simulink model "MOCS_AS_Gen"  (R2024b)
settings: Solver=FixedStepDiscrete  StartTime=0.0  StopTime=inf  FixedStep=SamplingTime  RelTol=1e-3
PostLoadFcn:
  | init_EXT_SRTUCT_IN;
model workspace: external: MAT-File (data not in the file)
undefined symbols (not defined in the file): IF_MATIN_IO, IF_PARA, IO_typ, Para_typ, Tick_100ms
libraries: simulink x10, bur_blks x3, Lib_Model x1
settings Model: DataDictionary=mainDB.sldd  Creator=HHI  LastModifiedBy=HHI
settings DataIOCC: SaveFormat=Array  SaveOutput=off  SignalLogging=off  DSMLogging=off  SaveTime=off  ReturnWorkspaceOutputs=off
settings OptimizationCC: ReuseModelBlockBuffer=off  EnableMemcpy=off  ZeroExternalMemoryAtStartup=off  ZeroInternalMemoryAtStartup=off  InitFltsAndDblsToZero=on  LifeSpan=inf  OptimizeBlockOrder=speed  DifferentSizesBufferReuse=on  EfficientTunableParamExpr=on
settings DebuggingCC: UnderspecifiedInitializationDetection=Classic  MergeDetectMultiDrivingBlocksExec=none  SolverPrmCheckMsg=warning  InheritedTsInSrcMsg=none  FcnCallInpInsideContextMsg=warning  UnconnectedInputMsg=warning  UnconnectedOutputMsg=warning  UnconnectedLineMsg=warning  FrameProcessingCompatibilityMsg=none  ModelReferenceSymbolNameMessage=none  StateNameClashWarn=warning  SFUnexpectedBacktrackingDiag=warning  SFNoUnconditionalDefaultTransitionDiag=warning
settings HardwareCC: ProdBitPerPointer=32  ProdBitPerSizeT=32  ProdBitPerPtrDiffT=32  ProdLargestAtomicFloat=None  ProdWordSize=32  ProdHWDeviceType=Intel->x86/Pentium
settings ModelReferenceCC: UpdateModelReferenceTargets=IfOutOfDate  ModelReferencePassRootInputsByReference=off  PropagateSignalLabelsOutOfModel=off
settings SFSimCC: MATLABDynamicMemAlloc=off
settings RTWCC: Description=B&R Automation Studio Target (ERT based)  SystemTargetFile=bur_ert.tlc  GenCodeOnly=on  GenerateMakefile=off  TemplateMakefile=bur.tmf  RTWVerbose=off  GPUComputeCapability=3.5
settings CodeAppCC: IgnoreTestpoints=on  CustomSymbolStrType=$N$R$M  InternalIdentifier=Classic
settings STFCustomTargetCC: TargetLangStandard=C99 (ISO)  MultiwordLength=256  ParMdlRefBuildCompliant=on  ERTCustomFileBanners=on  SupportNonFinite=off  SupportNonInlinedSFcns=off  RemoveResetFunc=on  MATLABClassNameForMDSCustomization=Simulink.SoftwareTarget.ERTCustomization  SystemTargetFile=bur_ert.tlc
settings ERTTargetCC: TargetLangStandard=C99 (ISO)  CompOptLevelCompliant=off  ConcurrentExecutionCompliant=off  CombineOutputUpdateFcns=off  SupportNonFinite=off  SupportContinuousTime=on  ModelStepFunctionPrototypeControlCompliant=off  CPPClassGenCompliant=off  UseToolchainInfoCompliant=off  ExtModeMexArgs='127.0.0.1'  InlinedParameterPlacement=Hierarchical  MultiInstanceErrorCode=Warning  RootIOFormat=Structure reference  ERTSrcFileBannerTemplate=bur_code_c_template.cgt  ERTHdrFileBannerTemplate=bur_code_h_template.cgt  ERTDataSrcFileTemplate=bur_data_c_template.cgt  ERTDataHdrFileTemplate=bur_data_h_template.cgt  ERTCustomFileTemplate=bur_file_process.tlc  ConvertIfToSwitch=off  SuppressUnreachableDefaultCases=off  DynamicArrayContainerType=coder::array

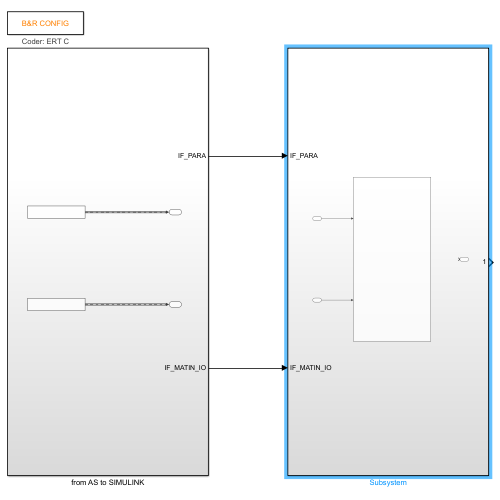
[thumbnail: Simulink's stored preview of the top-level diagram]
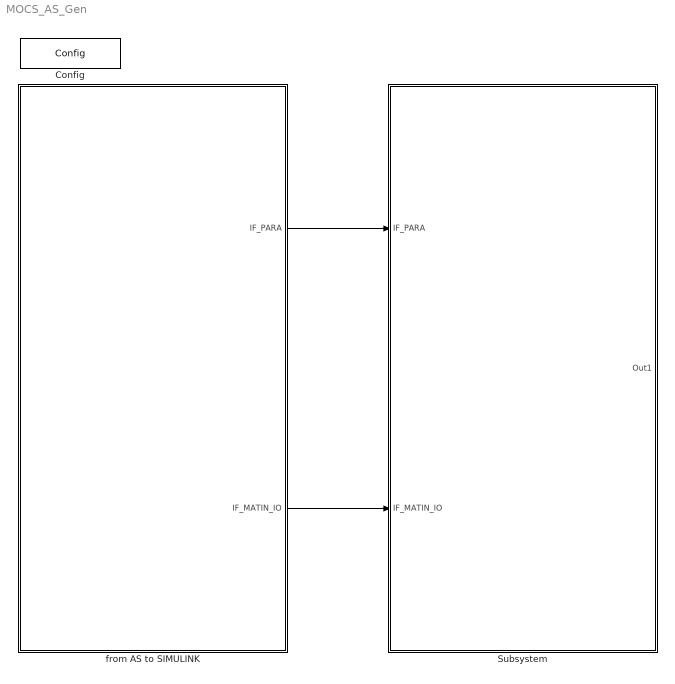
== system MOCS_AS_Gen ==
  Config : bur_blks/Config  Tag=Coder: ERT C Target: Task  bur_configset_ert=C - Code Generation (Embedded Real Time Target based)  bur_configset_grt=C - Code Generation (Generic Real Time Target based)  bur_maskHandle=-1
      settings: AttributesFormatString=%<Tag>  SourceProductName=B&R Automation Studio Toolbox
  Subsystem : Subsystem
  from AS to SIMULINK : Subsystem
  wires:
  from AS to SIMULINK/1(IF_PARA) -> Subsystem/1(IF_PARA)
  from AS to SIMULINK/2(IF_MATIN_IO) -> Subsystem/2(IF_MATIN_IO)

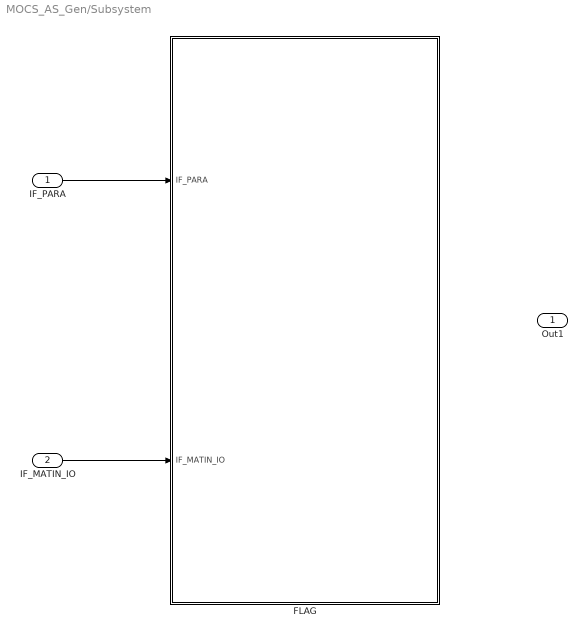
== system MOCS_AS_Gen/Subsystem ==
  IF_PARA : Inport
  IF_MATIN_IO : Inport  Port=2
  FLAG : Subsystem
  Out1 : Outport
  wires:
  IF_PARA/1 -> FLAG/1(IF_PARA)
  IF_MATIN_IO/1 -> FLAG/2(IF_MATIN_IO)

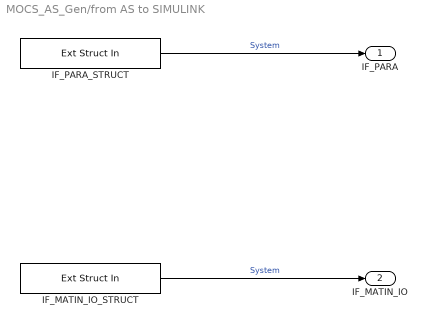
== system MOCS_AS_Gen/from AS to SIMULINK ==
  IF_MATIN_IO_STRUCT : bur_blks/Ext Struct In  Tag=GLOBAL IO_typ IF_MATIN_IO  bur_var_name=IF_MATIN_IO  bur_scope=GLOBAL  bur_var_memory=standard  bur_struct_name=IO_typ  bur_AS_string=IF_MATIN_IO : IO_typ; (**)  bur_AS_typ_list_string=|
      | IO_typ
      | Bus: CommIO_typ
      | Bus: CommMOCSIO_typ
      | Bus: CMDI_typ
      | Bus: CMDO_typ
      | Bus: CommFODSIO_typ
      | Bus: CFAI_typ
      | Bus: CFDI_typ
      | Bus: CFDO_typ
      | Bus: IndivIO_typ
      | Bus: IndivMOCSIO_typ
      | Bus: IMAI_typ
      | Bus: IMAO_typ
      | Bus: IMDI_typ
      | Bus: IMDO_typ
      | Bus: IndivFODSIO_typ
      | Bus: IFAI_typ
      | Bus: IFAO_typ
      | Bus: IFDI_typ
      | Bus: IFDO_typ
      | Bus: IndivSCRIO_typ
      | Bus: ISDI_typ
      | Bus: ISDO_typ
      | Bus: IndivIO_typ
      | Bus: IndivMOCSIO_typ
      | Bus: IMAI_typ
      | Bus: IMAO_typ
      | Bus: IMDI_typ
      | Bus: IMDO_typ
      | Bus: IndivFODSIO_typ
      | Bus: IFAI_typ
      | Bus: IFAO_typ
      | Bus: IFDI_typ
      | Bus: IFDO_typ
      | Bus: IndivSCRIO_typ
      | Bus: ISDI_typ
      | Bus: ISDO_typ
      | Bus: IndivIO_typ
      | Bus: IndivMOCSIO_typ
      | Bus: IMAI_typ
      | Bus: IMAO_typ
      | Bus: IMDI_typ
      | Bus: IMDO_typ
      | Bus: IndivFODSIO_typ
      | Bus: IFAI_typ
      | Bus: IFAO_typ
      | Bus: IFDI_typ
      | Bus: IFDO_typ
      | Bus: IndivSCRIO_typ
      | Bus: ISDI_typ
      | Bus: ISDO_typ
      | Bus: IndivIO_typ
      | Bus: IndivMOCSIO_typ
      | Bus: IMAI_typ
      | Bus: IMAO_typ
      | Bus: IMDI_typ
      | Bus: IMDO_typ
      | Bus: IndivFODSIO_typ
      | Bus: IFAI_typ
      | Bus: IFAO_typ
      | Bus: IFDI_typ
      | Bus: IFDO_typ
      | Bus: IndivSCRIO_typ
      | Bus: ISDI_typ
      | Bus: ISDO_typ
      | Bus: IndivIO_typ
      | Bus: IndivMOCSIO_typ
      | Bus: IMAI_typ
      | Bus: IMAO_typ
      | Bus: IMDI_typ
      | Bus: IMDO_typ
      | Bus: IndivFODSIO_typ
      | Bus: IFAI_typ
      | Bus: IFAO_typ
      | Bus: IFDI_typ
      | Bus: IFDO_typ
      | Bus: IndivSCRIO_typ
      | Bus: ISDI_typ
      | Bus: ISDO_typ
      | Bus: IndivIO_typ
      | Bus: IndivMOCSIO_typ
      | Bus: IMAI_typ
      | Bus: IMAO_typ
      | Bus: IMDI_typ
      | Bus: IMDO_typ
      | Bus: IndivFODSIO_typ
      | Bus: IFAI_typ
      | Bus: IFAO_typ
      | Bus: IFDI_typ
      | Bus: IFDO_typ
      | Bus: IndivSCRIO_typ
      | Bus: ISDI_typ
      | Bus: ISDO_typ
      | Bus: IndivIO_typ
      | Bus: IndivMOCSIO_typ
      | Bus: IMAI_typ
      | Bus: IMAO_typ
      | Bus: IMDI_typ
      | Bus: IMDO_typ
      | Bus: IndivFODSIO_typ
      | Bus: IFAI_typ
      | Bus: IFAO_typ
      | Bus: IFDI_typ
      | Bus: IFDO_typ
      | Bus: IndivSCRIO_typ
      | Bus: ISDI_typ
      | Bus: ISDO_typ
      | Bus: IndivIO_typ
      | Bus: IndivMOCSIO_typ
      | Bus: IMAI_typ
      | Bus: IMAO_typ
      | Bus: IMDI_typ
      | Bus: IMDO_typ
      | Bus: IndivFODSIO_typ
      | Bus: IFAI_typ
      | Bus: IFAO_typ
      | Bus: IFDI_typ
      | Bus: IFDO_typ
      | Bus: IndivSCRIO_typ
      | Bus: ISDI_typ
      | Bus: ISDO_typ
      settings: AttributesFormatString=%<Tag>  SourceProductName=B&R Automation Studio Toolbox
  IF_PARA_STRUCT : bur_blks/Ext Struct In  Tag=GLOBAL Para_typ IF_PARA  bur_var_name=IF_PARA  bur_scope=GLOBAL  bur_var_memory=standard  bur_struct_name=Para_typ  bur_AS_string=IF_PARA : Para_typ; (**)  bur_AS_typ_list_string=|
      | Para_typ
      | Bus: ParaCommon_typ
      | Bus: System_typ
      | Bus: SystemType_typ
      | Bus: SystemReserved_typ
      | Bus: StateFlag_typ
      | Bus: MSSNormalFlag_typ
      | Bus: LoadChangeFlag_typ
      | Bus: SystemWarmedUpFlag_typ
      | Bus: TMBFlag_typ
      | Bus: FlagReserved_typ
      | Bus: Main_typ
      | Bus: Init_typ
      | Bus: Sealing_typ
      | Bus: Engage_typ
      | Bus: Active_typ
      | Bus: TMB_typ
      | Bus: Disengage_typ
      | Bus: Airventing_typ
      | Bus: MOCSshutdown_typ
      | Bus: Valveshutdown_typ
      | Bus: FODS_typ
      | Bus: FODSInitReady_typ
      | Bus: FODSCooling_typ
      | Bus: FODSDosing_typ
      | Bus: FODSFlushing_typ
      | Bus: CommonReservedCat2_typ
      | Bus: CommonReservedCat3_typ
      | Bus: ParaIndiv_typ
      | Bus: FODSFeedforward_typ
      | Bus: FFpara_typ
      | Bus: EngineLoad_typ
      | Bus: ExhFlowrate_typ
      | Bus: HUInletRefTemp_typ
      | Bus: CorrectionFactor_typ
      | Bus: FODSFeedback_typ
      | Bus: MOCSTempPgain_typ
      | Bus: APIDgain_typ
      | Bus: IndivReservedCat2_typ
      | Bus: IndivReservedCat3_typ
      | Bus: ParaIndiv_typ
      | Bus: FODSFeedforward_typ
      | Bus: FFpara_typ
      | Bus: EngineLoad_typ
      | Bus: ExhFlowrate_typ
      | Bus: HUInletRefTemp_typ
      | Bus: CorrectionFactor_typ
      | Bus: FODSFeedback_typ
      | Bus: MOCSTempPgain_typ
      | Bus: APIDgain_typ
      | Bus: IndivReservedCat2_typ
      | Bus: IndivReservedCat3_typ
      | Bus: ParaIndiv_typ
      | Bus: FODSFeedforward_typ
      | Bus: FFpara_typ
      | Bus: EngineLoad_typ
      | Bus: ExhFlowrate_typ
      | Bus: HUInletRefTemp_typ
      | Bus: CorrectionFactor_typ
      | Bus: FODSFeedback_typ
      | Bus: MOCSTempPgain_typ
      | Bus: APIDgain_typ
      | Bus: IndivReservedCat2_typ
      | Bus: IndivReservedCat3_typ
      | Bus: ParaIndiv_typ
      | Bus: FODSFeedforward_typ
      | Bus: FFpara_typ
      | Bus: EngineLoad_typ
      | Bus: ExhFlowrate_typ
      | Bus: HUInletRefTemp_typ
      | Bus: CorrectionFactor_typ
      | Bus: FODSFeedback_typ
      | Bus: MOCSTempPgain_typ
      | Bus: APIDgain_typ
      | Bus: IndivReservedCat2_typ
      | Bus: IndivReservedCat3_typ
      | Bus: ParaIndiv_typ
      | Bus: FODSFeedforward_typ
      | Bus: FFpara_typ
      | Bus: EngineLoad_typ
      | Bus: ExhFlowrate_typ
      | Bus: HUInletRefTemp_typ
      | Bus: CorrectionFactor_typ
      | Bus: FODSFeedback_typ
      | Bus: MOCSTempPgain_typ
      | Bus: APIDgain_typ
      | Bus: IndivReservedCat2_typ
      | Bus: IndivReservedCat3_typ
      | Bus: ParaIndiv_typ
      | Bus: FODSFeedforward_typ
      | Bus: FFpara_typ
      | Bus: EngineLoad_typ
      | Bus: ExhFlowrate_typ
      | Bus: HUInletRefTemp_typ
      | Bus: CorrectionFactor_typ
      | Bus: FODSFeedback_typ
      | Bus: MOCSTempPgain_typ
      | Bus: APIDgain_typ
      | Bus: IndivReservedCat2_typ
      | Bus: IndivReservedCat3_typ
      | Bus: ParaIndiv_typ
      | Bus: FODSFeedforward_typ
      | Bus: FFpara_typ
      | Bus: EngineLoad_typ
      | Bus: ExhFlowrate_typ
      | Bus: HUInletRefTemp_typ
      | Bus: CorrectionFactor_typ
      | Bus: FODSFeedback_typ
      | Bus: MOCSTempPgain_typ
      | Bus: APIDgain_typ
      | Bus: IndivReservedCat2_typ
      | Bus: IndivReservedCat3_typ
      | Bus: ParaIndiv_typ
      | Bus: FODSFeedforward_typ
      | Bus: FFpara_typ
      | Bus: EngineLoad_typ
      | Bus: ExhFlowrate_typ
      | Bus: HUInletRefTemp_typ
      | Bus: CorrectionFactor_typ
      | Bus: FODSFeedback_typ
      | Bus: MOCSTempPgain_typ
      | Bus: APIDgain_typ
      | Bus: IndivReservedCat2_typ
      | Bus: IndivReservedCat3_typ
      settings: AttributesFormatString=%<Tag>  SourceProductName=B&R Automation Studio Toolbox
  IF_PARA : Outport
  IF_MATIN_IO : Outport  Port=2
  wires:
  IF_MATIN_IO_STRUCT/1 -> IF_MATIN_IO/1  "System"
  IF_PARA_STRUCT/1 -> IF_PARA/1  "System"

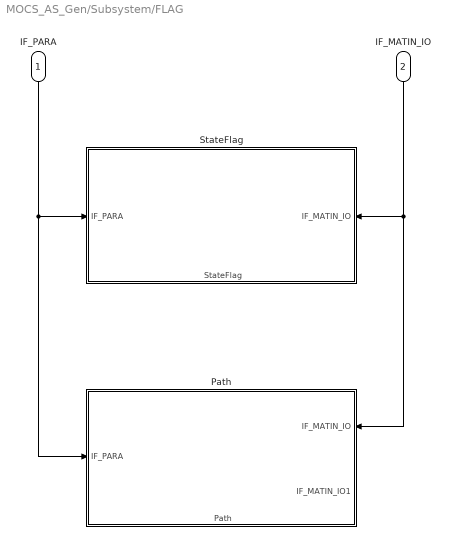
== system MOCS_AS_Gen/Subsystem/FLAG ==
  IF_PARA : Inport
  IF_MATIN_IO : Inport  Port=2
  Path : Subsystem
      settings: PortSchema="{\"entries\":[{\"content\":{\"sides\":[{\"content\":{\"connectorIds\":[\"In1\"]},\"type\":\"ConnectorPlacement.EquallySpacedRectSide\",\"uuid\":\"1f318d8d-d3a5-4a2a-9b6b-9d175d0730d5\"},{\"content\":{\"connectorIds\":[\"In2\",\"In3\"],\"side\":\"RIGHT\"},\"type\":\"ConnectorPlacement.EquallySpacedRectSide\",\"uuid\":\"3adb6d5c-76f6-48ff-b596-6c67523adb18\"},{\"content\":{\"side\":\"TOP\"},\"type\":\"ConnectorPlacement.EquallySpacedRectSide\",\"uuid\":\"8e39d891-14ef-4b5d-bc89-d43298abfc6f\"},{\"content\":{\"connectorIds\":[\"Out1\"],\"side\":\"BOTTOM\"},\"type\":\"ConnectorPlacement.EquallySpacedRectSide\",\"uuid\":\"e469beb5-ea4e-4c11-97b4-1468e014fe2c\"}]},\"type\":\"ConnectorPlacement.EquallySpacedConnector\",\"uuid\":\"bc676d84-16bc-4c83-9fee-587d58932695\"}],\"packageUris\":[\"http://schema.mathworks.com/mf0/Connector/R2020b\"],\"version\":\"1.0\"}"
  StateFlag : Subsystem
      settings: PortSchema="{\"entries\":[{\"content\":{\"sides\":[{\"content\":{\"connectorIds\":[\"In1\"]},\"type\":\"ConnectorPlacement.EquallySpacedRectSide\",\"uuid\":\"1f318d8d-d3a5-4a2a-9b6b-9d175d0730d5\"},{\"content\":{\"connectorIds\":[\"In2\"],\"side\":\"RIGHT\"},\"type\":\"ConnectorPlacement.EquallySpacedRectSide\",\"uuid\":\"3adb6d5c-76f6-48ff-b596-6c67523adb18\"},{\"content\":{\"side\":\"TOP\"},\"type\":\"ConnectorPlacement.EquallySpacedRectSide\",\"uuid\":\"8e39d891-14ef-4b5d-bc89-d43298abfc6f\"},{\"content\":{\"connectorIds\":[\"Out1\"],\"side\":\"BOTTOM\"},\"type\":\"ConnectorPlacement.EquallySpacedRectSide\",\"uuid\":\"a3ab5608-36e7-4443-b9c4-43378f0893dc\"}]},\"type\":\"ConnectorPlacement.EquallySpacedConnector\",\"uuid\":\"bc676d84-16bc-4c83-9fee-587d58932695\"}],\"packageUris\":[\"http://schema.mathworks.com/mf0/Connector/R2020b\"],\"version\":\"1.0\"}"
  wires:
  IF_MATIN_IO/1 -> StateFlag/2(IF_MATIN_IO), Path/2(IF_MATIN_IO)
  IF_PARA/1 -> Path/1(IF_PARA), StateFlag/1(IF_PARA)

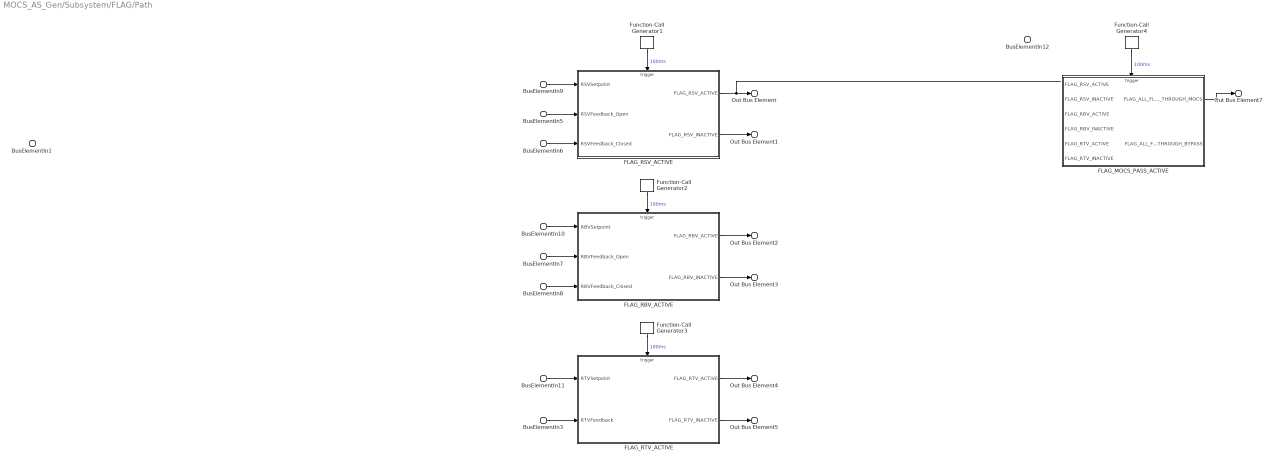
== system MOCS_AS_Gen/Subsystem/FLAG/Path ==
  BusElementIn1 : Inport  PortName=IF_PARA
  BusElementIn3 : Inport  Port=2  PortName=IF_MATIN_IO  Element=No1.MOCS.AIPro.RTVFeedback
  BusElementIn5 : Inport  Port=2  PortName=IF_MATIN_IO  Element=No1.MOCS.DIPro.RSVFeedback_Open
  BusElementIn6 : Inport  Port=2  PortName=IF_MATIN_IO  Element=No1.MOCS.DIPro.RSVFeedback_Closed
  BusElementIn7 : Inport  Port=2  PortName=IF_MATIN_IO  Element=No1.MOCS.DIPro.RBVFeedback_Open
  BusElementIn8 : Inport  Port=2  PortName=IF_MATIN_IO  Element=No1.MOCS.DIPro.RBVFeedback_Closed
  BusElementIn9 : Inport  Port=2  PortName=IF_MATIN_IO  Element=No1.MOCS.DOPro.RSVSetpoint
  BusElementIn10 : Inport  Port=2  PortName=IF_MATIN_IO  Element=No1.MOCS.DOPro.RBVSetpoint
  BusElementIn11 : Inport  Port=2  PortName=IF_MATIN_IO  Element=No1.MOCS.AOPro.RTVSetpoint
  BusElementIn12 : Inport  Port=3  PortName=IF_MATIN_IO1  Element=No1.MOCS.DOPro.RSVSetpoint
  FLAG_MOCS_PASS_ACTIVE : Stateflow chart  TreatAsAtomicUnit=on
  FLAG_RBV_ACTIVE : Stateflow chart  TreatAsAtomicUnit=on
  FLAG_RSV_ACTIVE : Stateflow chart  TreatAsAtomicUnit=on
  FLAG_RTV_ACTIVE : Stateflow chart  TreatAsAtomicUnit=on
  Function-Call Generator{1..4} (4 alike) : simulink/Ports & Subsystems/Function-Call Generator  sample_time=1/Tick_100ms  numberOfIterations=1  DisallowWideOutput=off
  Out Bus Element : Outport  PortName=Path  Element=RSV_ACTIVE
  Out Bus Element1 : Outport  PortName=Path  Element=RSV_INACTIVE
  Out Bus Element2 : Outport  PortName=Path  Element=RBV_ACTIVE
  Out Bus Element3 : Outport  PortName=Path  Element=RBV_INACTIVE
  Out Bus Element4 : Outport  PortName=Path  Element=RTV_ACTIVE
  Out Bus Element5 : Outport  PortName=Path  Element=RTV_INACTIVE
  Out Bus Element7 : Outport  PortName=Path  Element=FLAG_MOCS_PASS_ACTIVE
  wires:
  Function-Call Generator1/1 -> FLAG_RSV_ACTIVE/Trigger  "100ms"
  BusElementIn9/1 -> FLAG_RSV_ACTIVE/1(RSVSetpoint)
  BusElementIn5/1 -> FLAG_RSV_ACTIVE/2(RSVFeedback_Open)
  BusElementIn6/1 -> FLAG_RSV_ACTIVE/3(RSVFeedback_Closed)
  Function-Call Generator2/1 -> FLAG_RBV_ACTIVE/Trigger  "100ms"
  BusElementIn7/1 -> FLAG_RBV_ACTIVE/2(RBVFeedback_Open)
  BusElementIn8/1 -> FLAG_RBV_ACTIVE/3(RBVFeedback_Closed)
  BusElementIn10/1 -> FLAG_RBV_ACTIVE/1(RBVSetpoint)
  Function-Call Generator3/1 -> FLAG_RTV_ACTIVE/Trigger  "100ms"
  BusElementIn3/1 -> FLAG_RTV_ACTIVE/2(RTVFeedback)
  BusElementIn11/1 -> FLAG_RTV_ACTIVE/1(RTVSetpoint)
  FLAG_RSV_ACTIVE/2(FLAG_RSV_INACTIVE) -> Out Bus Element1/1
  FLAG_RBV_ACTIVE/1(FLAG_RBV_ACTIVE) -> Out Bus Element2/1
  FLAG_RTV_ACTIVE/1(FLAG_RTV_ACTIVE) -> Out Bus Element4/1
  FLAG_MOCS_PASS_ACTIVE/1(FLAG_ALL_FLOW_THROUGH_MOCS) -> Out Bus Element7/1
  FLAG_RTV_ACTIVE/2(FLAG_RTV_INACTIVE) -> Out Bus Element5/1
  FLAG_RBV_ACTIVE/2(FLAG_RBV_INACTIVE) -> Out Bus Element3/1
  FLAG_RSV_ACTIVE/1(FLAG_RSV_ACTIVE) -> Out Bus Element/1
  Function-Call Generator4/1 -> FLAG_MOCS_PASS_ACTIVE/Trigger  "100ms"

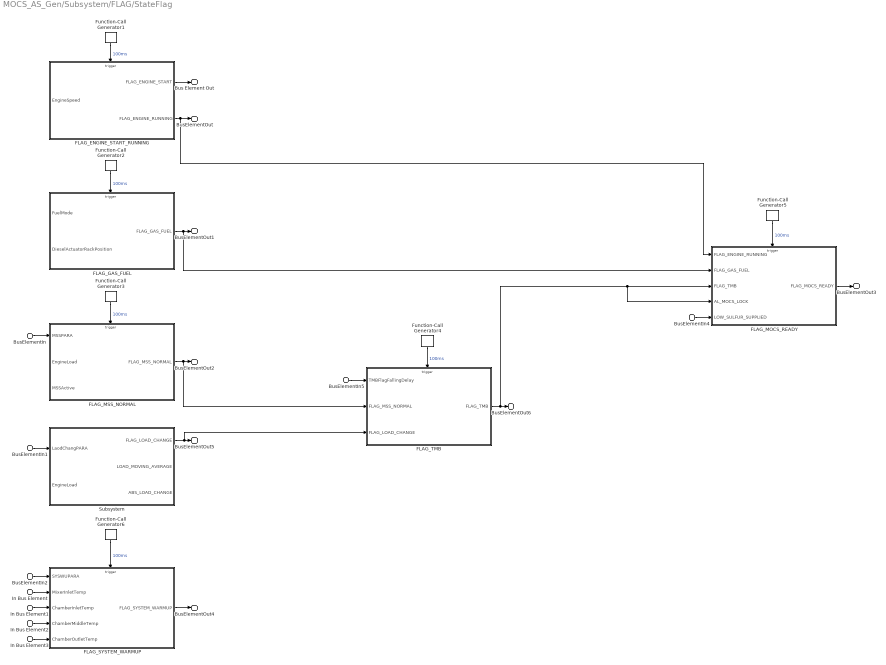
== system MOCS_AS_Gen/Subsystem/FLAG/StateFlag ==
  BusElementIn : Inport  PortName=IF_PARA  Element=Common.StateFlag.MSSNormalFlag
  BusElementIn1 : Inport  PortName=IF_PARA  Element=Common.StateFlag.LoadChangeFlag
  BusElementIn2 : Inport  PortName=IF_PARA  Element=Common.StateFlag.SystemWarmedUpFlag
  BusElementIn5 : Inport  PortName=IF_PARA  Element=Common.StateFlag.TMBFlag.TMBFlagFallingDelay
  In Bus Element : Inport  Port=2  PortName=IF_MATIN_IO  Element=No1.MOCS.AIPro.MixerInletTemp
  In Bus Element1 : Inport  Port=2  PortName=IF_MATIN_IO  Element=No1.MOCS.AIPro.ChamberInletTemp
  In Bus Element2 : Inport  Port=2  PortName=IF_MATIN_IO  Element=No1.MOCS.AIPro.ChamberMiddleTemp
  In Bus Element3 : Inport  Port=2  PortName=IF_MATIN_IO  Element=No1.MOCS.AIPro.ChamberOutletTemp
  BusElementIn4 : Inport  Port=2  PortName=IF_MATIN_IO  Element=No1.MOCS.DIPro.GELowSulfurfuelsupplied
  FLAG_ENGINE_START_RUNNING : Stateflow chart  TreatAsAtomicUnit=on
  FLAG_GAS_FUEL : Stateflow chart  TreatAsAtomicUnit=on
  FLAG_MOCS_READY : Stateflow chart  TreatAsAtomicUnit=on
  FLAG_MSS_NORMAL : Stateflow chart  TreatAsAtomicUnit=on
  FLAG_SYSTEM_WARMUP : Stateflow chart  TreatAsAtomicUnit=on
  FLAG_TMB : Stateflow chart  TreatAsAtomicUnit=on
  Function-Call Generator{1..6} (6 alike) : simulink/Ports & Subsystems/Function-Call Generator  sample_time=1/Tick_100ms  numberOfIterations=1  DisallowWideOutput=off
  Subsystem : Subsystem
  Bus Element Out : Outport  PortName=StateFlag  Element=ENGINE_START
  BusElementOut : Outport  PortName=StateFlag  Element=ENGINE_RUNNING
  BusElementOut1 : Outport  PortName=StateFlag  Element=GAS_FUEL
  BusElementOut2 : Outport  PortName=StateFlag  Element=MSS_NORMAL
  BusElementOut5 : Outport  PortName=StateFlag  Element=LOAD_CHANGE
  BusElementOut6 : Outport  PortName=StateFlag  Element=TMB
  BusElementOut3 : Outport  PortName=StateFlag  Element=MOCS_READY
  BusElementOut4 : Outport  PortName=StateFlag  Element=SYSTEM_WARMUP
  wires:
  Function-Call Generator1/1 -> FLAG_ENGINE_START_RUNNING/Trigger  "100ms"
  Function-Call Generator2/1 -> FLAG_GAS_FUEL/Trigger  "100ms"
  Function-Call Generator3/1 -> FLAG_MSS_NORMAL/Trigger  "100ms"
  BusElementIn1/1 -> Subsystem/1(LaodChangPARA)
  Function-Call Generator4/1 -> FLAG_TMB/Trigger  "100ms"
  Subsystem/1(FLAG_LOAD_CHANGE) -> BusElementOut5/1, FLAG_TMB/3(FLAG_LOAD_CHANGE)
  FLAG_MSS_NORMAL/1(FLAG_MSS_NORMAL) -> BusElementOut2/1, FLAG_TMB/2(FLAG_MSS_NORMAL)
  Function-Call Generator5/1 -> FLAG_MOCS_READY/Trigger  "100ms"
  Function-Call Generator6/1 -> FLAG_SYSTEM_WARMUP/Trigger  "100ms"
  BusElementIn4/1 -> FLAG_MOCS_READY/5(LOW_SULFUR_SUPPLIED)
  FLAG_ENGINE_START_RUNNING/2(FLAG_ENGINE_RUNNING) -> BusElementOut/1, FLAG_MOCS_READY/1(FLAG_ENGINE_RUNNING)
  FLAG_GAS_FUEL/1(FLAG_GAS_FUEL) -> FLAG_MOCS_READY/2(FLAG_GAS_FUEL), BusElementOut1/1
  FLAG_TMB/1(FLAG_TMB) -> BusElementOut6/1, FLAG_MOCS_READY/4(AL_MOCS_LOCK), FLAG_MOCS_READY/3(FLAG_TMB)
  BusElementIn2/1 -> FLAG_SYSTEM_WARMUP/1(SYSWUPARA)
  In Bus Element/1 -> FLAG_SYSTEM_WARMUP/2(MixerInletTemp)
  In Bus Element1/1 -> FLAG_SYSTEM_WARMUP/3(ChamberInletTemp)
  In Bus Element2/1 -> FLAG_SYSTEM_WARMUP/4(ChamberMiddleTemp)
  In Bus Element3/1 -> FLAG_SYSTEM_WARMUP/5(ChamberOutletTemp)
  BusElementIn/1 -> FLAG_MSS_NORMAL/1(MSSPARA)
  BusElementIn5/1 -> FLAG_TMB/1(TMBFlagFallingDelay)
  FLAG_ENGINE_START_RUNNING/1(FLAG_ENGINE_START) -> Bus Element Out/1
  FLAG_MOCS_READY/1(FLAG_MOCS_READY) -> BusElementOut3/1
  FLAG_SYSTEM_WARMUP/1(FLAG_SYSTEM_WARMUP) -> BusElementOut4/1

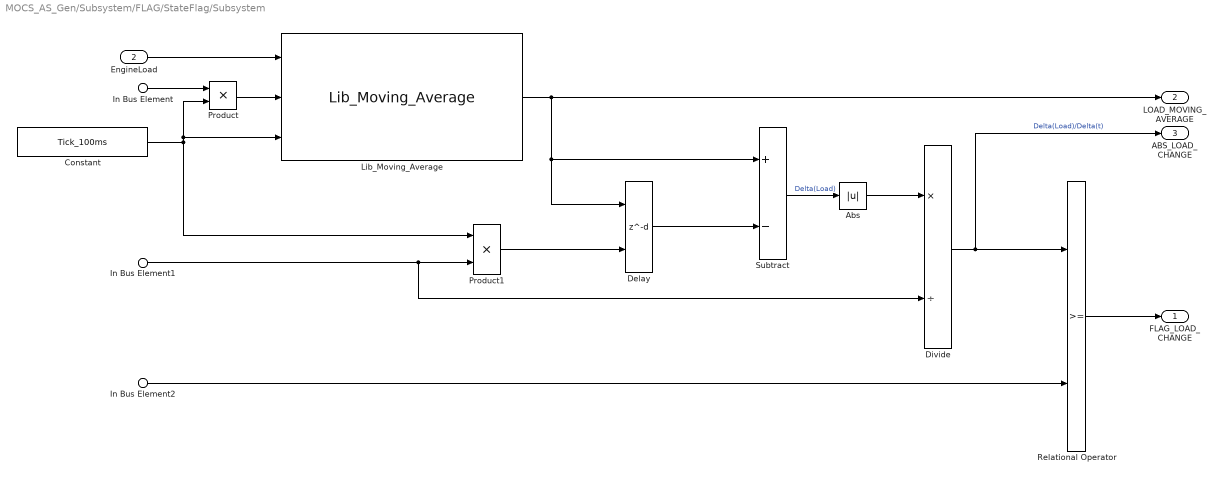
== system MOCS_AS_Gen/Subsystem/FLAG/StateFlag/Subsystem ==
  In Bus Element : Inport  PortName=LaodChangPARA  Element=MovAvgPeriod
  In Bus Element1 : Inport  PortName=LaodChangPARA  Element=ComparePoint
  In Bus Element2 : Inport  PortName=LaodChangPARA  Element=LoadChangeThreshold
  EngineLoad : Inport  Port=2
  Abs : Abs  SaturateOnIntegerOverflow=off
  Constant : Constant  Value=Tick_100ms
  Delay : Delay  DelayLengthSource=Input port
      settings: InputPortMap=u0,p1
  Divide : Product  Inputs=*/
  Lib_Moving_Average : Lib_Model/Lib_Moving_Average  SystemSampleTime=-1  VariantActivationTime=update diagram  AllowFlexibleInterface=on  Latency=0  AutoFrameSizeCalculation=off
  Product : Product
  Product1 : Product
  Relational Operator : RelationalOperator  OutDataTypeStr=boolean  RndMeth=Simplest  InputSameDT=off
  Subtract : Sum  Inputs=+-
  FLAG_LOAD_CHANGE : Outport
  LOAD_MOVING_AVERAGE : Outport  Port=2
  ABS_LOAD_CHANGE : Outport  Port=3
  wires:
  EngineLoad/1 -> Lib_Moving_Average/1
  Product/1 -> Lib_Moving_Average/2
  In Bus Element/1 -> Product/1
  Constant/1 -> Lib_Moving_Average/3, Product/2, Product1/1
  Lib_Moving_Average/1 -> Delay/1, Subtract/1, LOAD_MOVING_AVERAGE/1
  Product1/1 -> Delay/2
  In Bus Element1/1 -> Product1/2, Divide/2
  Delay/1 -> Subtract/2
  Subtract/1 -> Abs/1  "Delta(Load)"
  Abs/1 -> Divide/1
  In Bus Element2/1 -> Relational Operator/2
  Divide/1 -> ABS_LOAD_CHANGE/1, Relational Operator/1  "Delta(Load)/Delta(t)"
  Relational Operator/1 -> FLAG_LOAD_CHANGE/1

== stateflow chart MOCS_AS_Gen/Subsystem/FLAG/StateFlag/FLAG_MSS_NORMAL ==
  settings: executeAtInitialization=1
  state INIT
    en:
    FLAG_MSS_NORMAL = 0;
  state CHECK_FLAG
    state FLAG_OFF
      en:
      FLAG_MSS_NORMAL = 0;
    state DELAY
    state FLAG_ON
      en:
      FLAG_MSS_NORMAL = 1;
    (default) -> FLAG_OFF
    FLAG_OFF -> (junction 21) : [EngineLoad ...
        |      >= MSSPARA.MOCSMinEngineLoad]
    (junction 23) -> FLAG_OFF [order 2]
    (junction 29) -> FLAG_OFF [order 1] : [!(EngineLoad ...
        |      >= MSSPARA.MOCSMinEngineLoad)]
    DELAY -> FLAG_OFF [order 3] : after(MSSPARA.MSSNormalFallingDelay*Tick_100ms, TIMER)
    (junction 21) -> (junction 23) [order 2]
    (junction 21) -> FLAG_ON [order 1] : [EngineLoad ...
        |      >= MSSPARA.MOCSReadyEngineLoad]
    (junction 23) -> FLAG_ON [order 1] : [MSSActive]
    (junction 33) -> DELAY [order 2]
    DELAY -> FLAG_ON [order 1] : [MSSActive]
    DELAY -> FLAG_ON [order 2] : [!( EngineLoad ...
        |      <= (MSSPARA.MOCSReadyEngineLoad ...
        |           - MSSPARA.MSSNormalFallingHysteresis) )]
    (junction 29) -> (junction 31) [order 2]
    (junction 31) -> (junction 33) [order 1] : [EngineLoad ...
        |      <= (MSSPARA.MOCSReadyEngineLoad ...
        |           - MSSPARA.MSSNormalFallingHysteresis)]
    FLAG_ON -> (junction 29)
    (junction 31) -> FLAG_ON [order 2]
    (junction 33) -> FLAG_ON [order 1] : [MSSActive]
  (default) -> INIT
  INIT -> CHECK_FLAG
  data: MSSPARA input Bus: MSSNormalFlag_typ; FLAG_MSS_NORMAL output boolean size=1; EngineLoad input single size=1; MSSActive input single size=1; Tick_100ms parameter double size=1
  events: TIMER input FUNCTION_CALL_EVENT

== stateflow chart MOCS_AS_Gen/Subsystem/FLAG/StateFlag/FLAG_TMB ==
  settings: executeAtInitialization=1
  state INIT
    en:
    FLAG_TMB = 0;
  state CHECK_FLAG
    state FLAG_OFF
      en:
      FLAG_TMB = 0;
    state DELAY
    state FLAG_ON
      en:
      FLAG_TMB = 1;
    (default) -> FLAG_OFF
    FLAG_OFF -> FLAG_ON : [FLAG_MSS_NORMAL == 0 ...
        | || FLAG_LOAD_CHANGE == 1]
    DELAY -> FLAG_OFF [order 2] : after(TMBFlagFallingDelay*Tick_100ms, TIMER)
    FLAG_ON -> DELAY : [!(FLAG_MSS_NORMAL == 0 ...
        | || FLAG_LOAD_CHANGE == 1)]
    DELAY -> FLAG_ON [order 1] : [FLAG_MSS_NORMAL == 0 ...
        | || FLAG_LOAD_CHANGE == 1]
  (default) -> INIT
  INIT -> CHECK_FLAG
  data: TMBFlagFallingDelay input single; FLAG_TMB output boolean size=1; FLAG_MSS_NORMAL input boolean size=1; FLAG_LOAD_CHANGE input boolean size=1; Tick_100ms parameter double size=1
  events: TIMER input FUNCTION_CALL_EVENT

== stateflow chart MOCS_AS_Gen/Subsystem/FLAG/StateFlag/FLAG_MOCS_READY ==
  settings: executeAtInitialization=1
  state INIT
    en:
    FLAG_MOCS_READY = 0;
  state CHECK_FLAG
    state FLAG_OFF
      en:
      FLAG_MOCS_READY = 0;
    state DELAY
    state FLAG_ON
      en:
      FLAG_MOCS_READY = 1;
    (default) -> FLAG_OFF
    FLAG_OFF -> FLAG_ON : [FLAG_ENGINE_RUNNING == 1 ...
        | && FLAG_GAS_FUEL == 1 ...
        | && FLAG_TMB == 1 ...
        | && AL_MOCS_LOCK == 0 ...
        | && LOW_SULFUR_SUPPLIED == 1]
    DELAY -> FLAG_OFF [order 2] : after(2, TIMER)
    DELAY -> FLAG_ON [order 1] : [FLAG_ENGINE_RUNNING == 1 ...
        | && FLAG_GAS_FUEL == 1 ...
        | && FLAG_TMB == 1 ...
        | && AL_MOCS_LOCK == 0 ...
        | && LOW_SULFUR_SUPPLIED == 1]
    FLAG_ON -> DELAY : [!(FLAG_ENGINE_RUNNING == 1 ...
        | && FLAG_GAS_FUEL == 1 ...
        | && FLAG_TMB == 1 ...
        | && AL_MOCS_LOCK == 0 ...
        | && LOW_SULFUR_SUPPLIED == 1)]
  (default) -> INIT
  INIT -> CHECK_FLAG
  data: FLAG_ENGINE_RUNNING input boolean size=1; FLAG_GAS_FUEL input boolean size=1; FLAG_MOCS_READY output boolean size=1; FLAG_TMB input boolean size=1; AL_MOCS_LOCK input boolean size=1; LOW_SULFUR_SUPPLIED input boolean size=1
  events: TIMER input FUNCTION_CALL_EVENT

== stateflow chart MOCS_AS_Gen/Subsystem/FLAG/StateFlag/FLAG_SYSTEM_WARMUP ==
  settings: executeAtInitialization=1
  state INIT
    en:
    FLAG_SYSTEM_WARMUP = 0;
  state CHECK_FLAG
    state FLAG_OFF
      en:
      FLAG_SYSTEM_WARMUP = 0;
    state FLAG_ON
      en:
      FLAG_SYSTEM_WARMUP = 1;
    (default) -> FLAG_OFF
    FLAG_OFF -> FLAG_ON : [MixerInletTemp >= SYSWUPARA.WarmUpITemp ...
        | && ChamberInletTemp >= SYSWUPARA.WarmUpChITemp ...
        | && ChamberMiddleTemp >= SYSWUPARA.WarmUpChMTemp ...
        | && ChamberOutletTemp >= SYSWUPARA.WarmUpChOTemp ...
        | && fabs(MixerInletTemp - ChamberInletTemp) <= SYSWUPARA.WarmUpITemp]
    FLAG_ON -> FLAG_OFF : [!(MixerInletTemp >= SYSWUPARA.WarmUpITemp ...
        | && ChamberInletTemp >= SYSWUPARA.WarmUpChITemp ...
        | && ChamberMiddleTemp >= SYSWUPARA.WarmUpChMTemp ...
        | && ChamberOutletTemp >= SYSWUPARA.WarmUpChOTemp ...
        | && fabs(MixerInletTemp - ChamberInletTemp) <= SYSWUPARA.WarmUpITemp)]
  (default) -> INIT
  INIT -> CHECK_FLAG
  data: SYSWUPARA input Bus: SystemWarmedUpFlag_typ; FLAG_SYSTEM_WARMUP output boolean size=1; MixerInletTemp input single size=1; ChamberInletTemp input single size=1; ChamberMiddleTemp input single size=1; ChamberOutletTemp input single size=1
  events: TIMER input FUNCTION_CALL_EVENT

== stateflow chart MOCS_AS_Gen/Subsystem/FLAG/Path/FLAG_RSV_ACTIVE ==
  settings: sampleTime=SamplingTime  executeAtInitialization=1
  state INIT
    en:
    FLAG_RSV_ACTIVE = 0;
    FLAG_RSV_INACTIVE = 0;
    Lo_RSV_CLOSE = 1;
    Lo_RSV_OPEN = 0; // NORMAL OPEN
  state CHECK_FLAG
    state CHECK_FLAG_RSV_ACTIVE [parallel]
      settings: executionOrder=1
      state FLAG_OFF
        en:
        FLAG_RSV_ACTIVE = 0;
      state FLAG_ON
        en:
        FLAG_RSV_ACTIVE = 1;
      (default) -> CHECK_FLAG.CHECK_FLAG_RSV_ACTIVE.FLAG_OFF
      CHECK_FLAG.CHECK_FLAG_RSV_ACTIVE.FLAG_OFF -> CHECK_FLAG.CHECK_FLAG_RSV_ACTIVE.FLAG_ON : [RSVSetpoint == Lo_RSV_OPEN ...
          | && RSVFeedback_Open == 1]
      CHECK_FLAG.CHECK_FLAG_RSV_ACTIVE.FLAG_ON -> CHECK_FLAG.CHECK_FLAG_RSV_ACTIVE.FLAG_OFF : [!(RSVSetpoint == Lo_RSV_OPEN ...
          | && RSVFeedback_Open == 1)]
    state CHECK_FLAG_RSV_INACTIVE [parallel]
      settings: executionOrder=2
      state FLAG_OFF
        en:
        FLAG_RSV_INACTIVE = 0;
      state FLAG_ON
        en:
        FLAG_RSV_INACTIVE = 1;
      (default) -> CHECK_FLAG.CHECK_FLAG_RSV_INACTIVE.FLAG_OFF
      CHECK_FLAG.CHECK_FLAG_RSV_INACTIVE.FLAG_OFF -> CHECK_FLAG.CHECK_FLAG_RSV_INACTIVE.FLAG_ON : [RSVSetpoint == Lo_RSV_CLOSE ...
          | && RSVFeedback_Closed == 1]
      CHECK_FLAG.CHECK_FLAG_RSV_INACTIVE.FLAG_ON -> CHECK_FLAG.CHECK_FLAG_RSV_INACTIVE.FLAG_OFF : [!(RSVSetpoint == Lo_RSV_CLOSE ...
          | && RSVFeedback_Closed == 1)]
  (default) -> INIT
  INIT -> CHECK_FLAG
  data: FLAG_RSV_ACTIVE output boolean size=1; RSVSetpoint input boolean size=1; FLAG_RSV_INACTIVE output boolean size=1; RSVFeedback_Open input boolean size=1; RSVFeedback_Closed input boolean size=1; Lo_RSV_CLOSE local boolean size=1 =1; Lo_RSV_OPEN local boolean size=1 =0
  data RSVSetpoint settings: description=|
      | 0: OPEN
      | 1: CLSOE
      | 
      | NORMAL OPEN
  events: TIMER input FUNCTION_CALL_EVENT

== stateflow chart MOCS_AS_Gen/Subsystem/FLAG/Path/FLAG_RBV_ACTIVE ==
  settings: sampleTime=SamplingTime  executeAtInitialization=1
  state INIT
    en:
    FLAG_RBV_ACTIVE = 0;
    FLAG_RBV_INACTIVE = 0;
    Lo_RBV_CLOSE = 1;
    Lo_RBV_OPEN = 0; // NORMAL OPEN
  state CHECK_FLAG
    state CHECK_FLAG_RBV_ACTIVE [parallel]
      settings: executionOrder=1
      state FLAG_OFF
        en:
        FLAG_RBV_ACTIVE = 0;
      state FLAG_ON
        en:
        FLAG_RBV_ACTIVE = 1;
      (default) -> CHECK_FLAG.CHECK_FLAG_RBV_ACTIVE.FLAG_OFF
      CHECK_FLAG.CHECK_FLAG_RBV_ACTIVE.FLAG_OFF -> CHECK_FLAG.CHECK_FLAG_RBV_ACTIVE.FLAG_ON : [RBVSetpoint == Lo_RBV_OPEN ...
          | && RBVFeedback_Open == 1]
      CHECK_FLAG.CHECK_FLAG_RBV_ACTIVE.FLAG_ON -> CHECK_FLAG.CHECK_FLAG_RBV_ACTIVE.FLAG_OFF : [!(RBVSetpoint == Lo_RBV_OPEN ...
          | && RBVFeedback_Open == 1)]
    state CHECK_FLAG_RBV_INACTIVE [parallel]
      settings: executionOrder=2
      state FLAG_OFF
        en:
        FLAG_RBV_INACTIVE = 0;
      state FLAG_ON
        en:
        FLAG_RBV_INACTIVE = 1;
      (default) -> CHECK_FLAG.CHECK_FLAG_RBV_INACTIVE.FLAG_OFF
      CHECK_FLAG.CHECK_FLAG_RBV_INACTIVE.FLAG_OFF -> CHECK_FLAG.CHECK_FLAG_RBV_INACTIVE.FLAG_ON : [RBVSetpoint == Lo_RBV_CLOSE ...
          | && RBVFeedback_Closed == 1]
      CHECK_FLAG.CHECK_FLAG_RBV_INACTIVE.FLAG_ON -> CHECK_FLAG.CHECK_FLAG_RBV_INACTIVE.FLAG_OFF : [!(RBVSetpoint == Lo_RBV_CLOSE ...
          | && RBVFeedback_Closed == 1)]
  (default) -> INIT
  INIT -> CHECK_FLAG
  data: FLAG_RBV_ACTIVE output boolean size=1; RBVSetpoint input boolean size=1; FLAG_RBV_INACTIVE output boolean size=1; RBVFeedback_Open input boolean size=1; RBVFeedback_Closed input boolean size=1; Lo_RBV_OPEN local boolean size=1 =0; Lo_RBV_CLOSE local boolean size=1 =1
  data RBVSetpoint settings: description=|
      | 0: OPEN
      | 1: CLSOE
      | 
      | NORMAL OPEN
  events: TIMER input FUNCTION_CALL_EVENT

== stateflow chart MOCS_AS_Gen/Subsystem/FLAG/Path/FLAG_RTV_ACTIVE ==
  settings: sampleTime=SamplingTime  executeAtInitialization=1
  state INIT
    en:
    FLAG_RTV_ACTIVE = 0;
    FLAG_RTV_INACTIVE = 0;
    Lo_RTV_CLOSE = 5;
    Lo_RTV_OPEN = 100 - Lo_RTV_CLOSE;
  state CHECK_FLAG
    state CHECK_FLAG_RTV_ACTIVE [parallel]
      settings: executionOrder=1
      state FLAG_OFF
        en:
        FLAG_RTV_ACTIVE = 0;
      state FLAG_ON
        en:
        FLAG_RTV_ACTIVE = 1;
      (default) -> CHECK_FLAG.CHECK_FLAG_RTV_ACTIVE.FLAG_OFF
      CHECK_FLAG.CHECK_FLAG_RTV_ACTIVE.FLAG_OFF -> CHECK_FLAG.CHECK_FLAG_RTV_ACTIVE.FLAG_ON : [RTVSetpoint == 100 ...
          | && RTVFeedback >= Lo_RTV_OPEN]
      CHECK_FLAG.CHECK_FLAG_RTV_ACTIVE.FLAG_ON -> CHECK_FLAG.CHECK_FLAG_RTV_ACTIVE.FLAG_OFF : [!(RTVSetpoint == 100 ...
          | && RTVFeedback >= Lo_RTV_OPEN)]
    state CHECK_FLAG_RTV_INACTIVE [parallel]
      settings: executionOrder=2
      state FLAG_OFF
        en:
        FLAG_RTV_INACTIVE = 0;
      state FLAG_ON
        en:
        FLAG_RTV_INACTIVE = 1;
      (default) -> CHECK_FLAG.CHECK_FLAG_RTV_INACTIVE.FLAG_OFF
      CHECK_FLAG.CHECK_FLAG_RTV_INACTIVE.FLAG_OFF -> CHECK_FLAG.CHECK_FLAG_RTV_INACTIVE.FLAG_ON : [RTVSetpoint == 0 ...
          | && RTVFeedback <= Lo_RTV_CLOSE]
      CHECK_FLAG.CHECK_FLAG_RTV_INACTIVE.FLAG_ON -> CHECK_FLAG.CHECK_FLAG_RTV_INACTIVE.FLAG_OFF : [!(RTVSetpoint == 0 ...
          | && RTVFeedback <= Lo_RTV_CLOSE)]
  (default) -> INIT
  INIT -> CHECK_FLAG
  data: FLAG_RTV_ACTIVE output boolean size=1; RTVSetpoint input single size=1; FLAG_RTV_INACTIVE output boolean size=1; RTVFeedback input single size=1; Lo_RTV_OPEN local single size=1; Lo_RTV_CLOSE local single size=1
  events: TIMER input FUNCTION_CALL_EVENT

== stateflow chart MOCS_AS_Gen/Subsystem/FLAG/Path/FLAG_MOCS_PASS_ACTIVE ==
  settings: sampleTime=SamplingTime  executeAtInitialization=1
  state INIT
    en:
    FLAG_ALL_FLOW_THROUGH_MOCS = 0;
    FLAG_ALL_FLOW_THROUGH_BYPASS = 0;
  state CHECK_FLAG
    state CHECK_FLAG_ALL_FLOW_THROUGH_MOCS [parallel]
      settings: executionOrder=1
      state FLAG_OFF
        en:
        FLAG_ALL_FLOW_THROUGH_MOCS = 0;
      state FLAG_ON
        en:
        FLAG_ALL_FLOW_THROUGH_MOCS = 1;
      (default) -> CHECK_FLAG.CHECK_FLAG_ALL_FLOW_THROUGH_MOCS.FLAG_OFF
      CHECK_FLAG.CHECK_FLAG_ALL_FLOW_THROUGH_MOCS.FLAG_OFF -> CHECK_FLAG.CHECK_FLAG_ALL_FLOW_THROUGH_MOCS.FLAG_ON : [FLAG_RSV_ACTIVE == 1 ...
          | && FLAG_RBV_INACTIVE == 1 ...
          | && FLAG_RTV_ACTIVE == 1]
      CHECK_FLAG.CHECK_FLAG_ALL_FLOW_THROUGH_MOCS.FLAG_ON -> CHECK_FLAG.CHECK_FLAG_ALL_FLOW_THROUGH_MOCS.FLAG_OFF : [!(FLAG_RSV_ACTIVE == 1 ...
          | && FLAG_RBV_INACTIVE == 1 ...
          | && FLAG_RTV_ACTIVE == 1)]
    state CHECK_FLAG_ALL_FLOW_THROUGH_BYPAS [parallel]
      settings: executionOrder=2
      state FLAG_OFF
        en:
        FLAG_ALL_FLOW_THROUGH_BYPASS = 0;
      state FLAG_ON
        en:
        FLAG_ALL_FLOW_THROUGH_BYPASS = 1;
      (default) -> CHECK_FLAG.CHECK_FLAG_ALL_FLOW_THROUGH_BYPAS.FLAG_OFF
      CHECK_FLAG.CHECK_FLAG_ALL_FLOW_THROUGH_BYPAS.FLAG_OFF -> CHECK_FLAG.CHECK_FLAG_ALL_FLOW_THROUGH_BYPAS.FLAG_ON : [FLAG_RBV_ACTIVE == 1 ...
          | && (FLAG_RSV_INACTIVE == 1 ...
          |      || FLAG_RTV_INACTIVE == 1)]
      CHECK_FLAG.CHECK_FLAG_ALL_FLOW_THROUGH_BYPAS.FLAG_ON -> CHECK_FLAG.CHECK_FLAG_ALL_FLOW_THROUGH_BYPAS.FLAG_OFF : [!( FLAG_RBV_ACTIVE == 1 ...
          | && (FLAG_RSV_INACTIVE == 1 ...
          |      || FLAG_RTV_INACTIVE == 1) )]
  (default) -> INIT
  INIT -> CHECK_FLAG
  data: FLAG_RSV_ACTIVE input boolean size=1; FLAG_ALL_FLOW_THROUGH_MOCS output boolean size=1; FLAG_RSV_INACTIVE input boolean size=1; FLAG_RBV_ACTIVE input boolean size=1; FLAG_RBV_INACTIVE input boolean size=1; FLAG_RTV_ACTIVE input boolean size=1; FLAG_RTV_INACTIVE input boolean size=1; FLAG_ALL_FLOW_THROUGH_BYPASS output boolean size=1
  data FLAG_RSV_ACTIVE settings: description=|
      | 0: OPEN
      | 1: CLSOE
      | 
      | NORMAL OPEN
  data FLAG_RSV_INACTIVE settings: description=|
      | 0: OPEN
      | 1: CLSOE
      | 
      | NORMAL OPEN
  data FLAG_ALL_FLOW_THROUGH_BYPASS settings: description=|
      | 0: OPEN
      | 1: CLSOE
      | 
      | NORMAL OPEN
  events: TIMER input FUNCTION_CALL_EVENT

== stateflow chart MOCS_AS_Gen/Subsystem/FLAG/StateFlag/FLAG_ENGINE_START_RUNNING ==
  settings: sampleTime=SamplingTime  executeAtInitialization=1
  state INIT
    en:
    Lo_ENGINE_START_SPEED = 30;
    FLAG_ENGINE_START = 0;
    Lo_ENGINE_RUNNING_SPEED = 850;
    FLAG_ENGINE_RUNNING = 0;
  state CHECK_FLAG
    state CHECK_FLAG_ENGINE_START [parallel]
      settings: executionOrder=1
      state FLAG_OFF
        en:
        FLAG_ENGINE_START = 0;
      state FLAG_ON
        en:
        FLAG_ENGINE_START = 1;
      (default) -> CHECK_FLAG.CHECK_FLAG_ENGINE_START.FLAG_OFF
      CHECK_FLAG.CHECK_FLAG_ENGINE_START.FLAG_OFF -> CHECK_FLAG.CHECK_FLAG_ENGINE_START.FLAG_ON : [EngineSpeed >= Lo_ENGINE_START_SPEED]
      CHECK_FLAG.CHECK_FLAG_ENGINE_START.FLAG_ON -> CHECK_FLAG.CHECK_FLAG_ENGINE_START.FLAG_OFF : [!(EngineSpeed >= Lo_ENGINE_START_SPEED)]
    state CHECK_FLAG_ENGINE_RUNNING [parallel]
      settings: executionOrder=2
      state FLAG_OFF
        en:
        FLAG_ENGINE_RUNNING = 0;
      state FLAG_ON
        en:
        FLAG_ENGINE_RUNNING = 1;
      (default) -> CHECK_FLAG.CHECK_FLAG_ENGINE_RUNNING.FLAG_OFF
      CHECK_FLAG.CHECK_FLAG_ENGINE_RUNNING.FLAG_OFF -> CHECK_FLAG.CHECK_FLAG_ENGINE_RUNNING.FLAG_ON : [EngineSpeed >= Lo_ENGINE_RUNNING_SPEED]
      CHECK_FLAG.CHECK_FLAG_ENGINE_RUNNING.FLAG_ON -> CHECK_FLAG.CHECK_FLAG_ENGINE_RUNNING.FLAG_OFF : [!(EngineSpeed >= Lo_ENGINE_RUNNING_SPEED)]
  (default) -> INIT
  INIT -> CHECK_FLAG
  data: FLAG_ENGINE_START output boolean size=1; EngineSpeed input single size=1; Lo_ENGINE_START_SPEED local single size=1; FLAG_ENGINE_RUNNING output boolean size=1; Lo_ENGINE_RUNNING_SPEED local single size=1
  events: TIMER input FUNCTION_CALL_EVENT

== stateflow chart MOCS_AS_Gen/Subsystem/FLAG/StateFlag/FLAG_GAS_FUEL ==
  settings: executeAtInitialization=1
  state INIT
    en:
    FLAG_GAS_FUEL = 0;
    Lo_GAS_RACK_POSIOTION = 2;
    Lo_BLACKOUT = 0;
    Lo_BACKUP = 1;
    Lo_DIESEL = 2;
    Lo_GAS = 3;
    Lo_FUEL_SHARING = 4;
    Lo_GAS_MSS = 5;
  state CHECK_FLAG
    state FLAG_OFF
      en:
      FLAG_GAS_FUEL = 0;
    state FLAG_ON
      en:
      FLAG_GAS_FUEL = 1;
    (default) -> FLAG_OFF
    FLAG_OFF -> FLAG_ON : [(FuelMode == Lo_GAS || FuelMode == Lo_GAS_MSS) ...
        |  && DieselActuatorRackPosition <= Lo_GAS_RACK_POSIOTION]
    FLAG_ON -> FLAG_OFF : [!( (FuelMode == Lo_GAS || FuelMode == Lo_GAS_MSS) ...
        |  && DieselActuatorRackPosition <= Lo_GAS_RACK_POSIOTION )]
  (default) -> INIT
  INIT -> CHECK_FLAG
  data: FLAG_GAS_FUEL output boolean size=1; FuelMode input single size=1; Lo_BACKUP local single size=1; Lo_BLACKOUT local single size=1; Lo_DIESEL local single size=1; Lo_FUEL_SHARING local single; Lo_GAS local single size=1; Lo_GAS_MSS local single; DieselActuatorRackPosition input single size=1; Lo_GAS_RACK_POSIOTION local single size=1
  events: TIMER input FUNCTION_CALL_EVENT
